simulink model "Mode_AAI"  (R2022b)
settings: Solver=FixedStepAuto  StartTime=0.0  StopTime=10.0  FixedStep=1e-3  RelTol=1e-3  EnableMultiTasking=on
undefined symbols (not defined in the file): D0, D10, D11, D12, D13, D2, D4, D5, D6, D7, D8, D9, PTA0, PTA2, PTB23, PTB9, PTC16, PTC2, PTC3, PTC4, PTD0, PTD1, PTD2, PTD3
libraries: frdmk64flib x14
settings Model: ExtModeTrigDuration=5  Creator=sarahalabdulrazzak  LastModifiedBy=kavem
settings SolverCC: AlgebraicLoopSolver=TrustRegion
settings OptimizationCC: EnhancedBackFolding=on  PassReuseOutputArgsAs=Individual arguments  ZeroExternalMemoryAtStartup=off  ZeroInternalMemoryAtStartup=off  MaxStackSize=64  OptimizeBlockOrder=speed  DifferentSizesBufferReuse=on  OptimizationCustomize=off  EfficientTunableParamExpr=on
settings DebuggingCC: ParameterTunabilityLossMsg=error  UnconnectedInputMsg=warning  UnconnectedOutputMsg=warning  UnconnectedLineMsg=warning  SFMachineParentedDataDiag=warning
settings HardwareCC: ProdBitPerPointer=32  ProdBitPerSizeT=32  ProdBitPerPtrDiffT=32  ProdLargestAtomicInteger=Long  ProdLargestAtomicFloat=Double  ProdWordSize=32  ProdHWDeviceType=ARM Compatible->ARM Cortex
settings ModelReferenceCC: EnableRefExpFcnMdlSchedulingChecks=on
settings SFSimCC: MATLABDynamicMemAlloc=off
settings RTWCC: Description=Embedded Coder  SystemTargetFile=ert.tlc  HardwareBoard=NXP FRDM-K64F  TLCOptions="-aInlineSetEventsForThisBaseRateFcn=TLC_FALSE -aSuppressMultiTaskScheduler=TLC_FALSE  -aRateBasedStepFcn=0"  TemplateMakefile=ert_default_tmf  Toolchain=GNU Tools for ARM Embedded Processors
settings CodeAppCC: ForceParamTrailComments=on  IgnoreCustomStorageClasses=off  OperatorAnnotations=on  SimulinkDataObjDesc=on  SFDataObjDesc=on  InsertBlockDesc=on

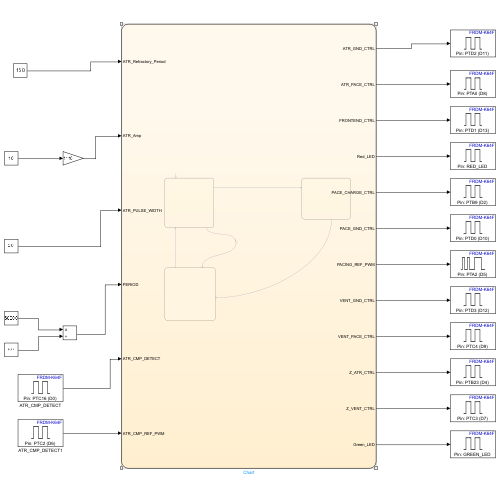
[thumbnail: Simulink's stored preview of the top-level diagram]
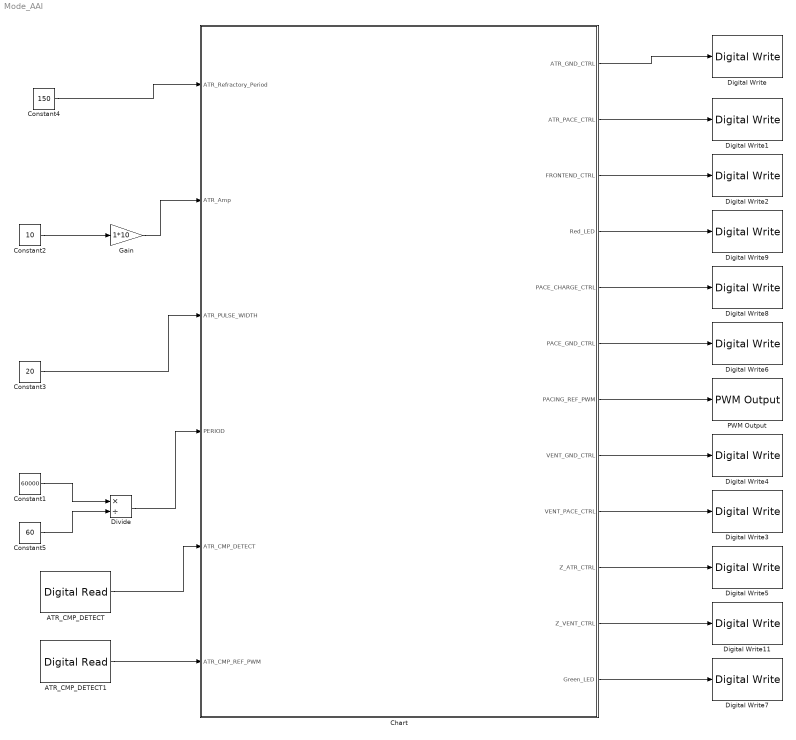
== system Mode_AAI ==
  ATR_CMP_DETECT : frdmk64flib/Digital Read  Whichpin=PTC16 (D0)  SampleTime=-1
  ATR_CMP_DETECT1 : frdmk64flib/Digital Read  Whichpin=PTC2 (D6)  SampleTime=-1
  Chart : Stateflow chart  TreatAsAtomicUnit=on
  Constant1 : Constant  Value=60000
  Constant2 : Constant  Value=10
  Constant3 : Constant  Value=20
  Constant4 : Constant  Value=150
  Constant5 : Constant  Value=60
  Digital Write : frdmk64flib/Digital Write  Whichpin=PTD2 (D11)
  Digital Write1 : frdmk64flib/Digital Write  Whichpin=PTA0 (D8)
  Digital Write11 : frdmk64flib/Digital Write  Whichpin=PTC3 (D7)
  Digital Write2 : frdmk64flib/Digital Write  Whichpin=PTD1 (D13)
  Digital Write3 : frdmk64flib/Digital Write  Whichpin=PTC4 (D9)
  Digital Write4 : frdmk64flib/Digital Write  Whichpin=PTD3 (D12)
  Digital Write5 : frdmk64flib/Digital Write  Whichpin=PTB23 (D4)
  Digital Write6 : frdmk64flib/Digital Write  Whichpin=PTD0 (D10)
  Digital Write7 : frdmk64flib/Digital Write  Whichpin=GREEN_LED
  Digital Write8 : frdmk64flib/Digital Write  Whichpin=PTB9 (D2)
  Digital Write9 : frdmk64flib/Digital Write  Whichpin=RED_LED
  Divide : Product  Inputs=*/
  Gain : Gain  Gain=1*10
  PWM Output : frdmk64flib/PWM Output  Whichpin=PTA2 (D5)  InitialFrequency=2000  InitialDutyCycle=0
  wires:
  Constant3/1 -> Chart/3(ATR_PULSE_WIDTH)
  Constant4/1 -> Chart/1(ATR_Refractory_Period)
  Chart/1(ATR_GND_CTRL) -> Digital Write/1
  Chart/2(ATR_PACE_CTRL) -> Digital Write1/1
  Chart/3(FRONTEND_CTRL) -> Digital Write2/1
  Chart/4(Red_LED) -> Digital Write9/1
  Chart/5(PACE_CHARGE_CTRL) -> Digital Write8/1
  Chart/6(PACE_GND_CTRL) -> Digital Write6/1
  Chart/7(PACING_REF_PWM) -> PWM Output/1
  Chart/8(VENT_GND_CTRL) -> Digital Write4/1
  Chart/9(VENT_PACE_CTRL) -> Digital Write3/1
  Chart/10(Z_ATR_CTRL) -> Digital Write5/1
  Chart/11(Z_VENT_CTRL) -> Digital Write11/1
  Constant5/1 -> Divide/2
  Constant1/1 -> Divide/1
  Divide/1 -> Chart/4(PERIOD)
  Constant2/1 -> Gain/1
  Gain/1 -> Chart/2(ATR_Amp)
  ATR_CMP_DETECT/1 -> Chart/5(ATR_CMP_DETECT)
  Chart/12(Green_LED) -> Digital Write7/1
  ATR_CMP_DETECT1/1 -> Chart/6(ATR_CMP_REF_PWM)

== stateflow chart Mode_AAI/Chart ==
  state CHARGING
    entry:
    %sensing ON
    FRONTEND_CTRL = HIGH
    %Charge primary capcitor C22
    ATR_PACE_CTRL=LOW
    VENT_PACE_CTRL=LOW
    PACING_REF_PWM = ATR_Amp
    PACE_CHARGE_CTRL = HIGH
    %Discharge block capacitor C21
    PACE_GND_CTRL = HIGH
    VENT_PACE_CTRL = LOW
    Z_ATR_CTRL = LOW
    Z_VENT_CTRL = LOW
    ATR_GND_CTRL = HIGH
    VENT_GND_CTRL = LOW
    %use LED  to verify state
    Red_LED=false
    Green_LED=true
  state DISCHARGING
    %sensing OFF
    FRONTEND_CTRL = LOW
    %Discharge C22 primary capacitor
    %Charge C21 block capacitor
    PACE_CHARGE_CTRL = LOW
    PACE_GND_CTRL = HIGH
    ATR_PACE_CTRL = HIGH
    ATR_GND_CTRL = LOW
    Z_ATR_CTRL = LOW
    Z_VENT_CTRL = LOW
    VENT_GND_CTRL = LOW
    VENT_PACE_CTRL  = LOW
    PACING_REF_PWM = ATR_Amp
    %use LED  to verify state
    Red_LED=true
  state STATE
    entry:
    %sensing ON
    FRONTEND_CTRL = LOW
    %Charge primary capcitor C22
    ATR_PACE_CTRL=LOW
    VENT_PACE_CTRL=LOW
    PACING_REF_PWM = ATR_Amp
    PACE_CHARGE_CTRL = HIGH
    %Discharge block capacitor C21
    PACE_GND_CTRL = HIGH
    VENT_PACE_CTRL = LOW
    Z_ATR_CTRL = LOW
    Z_VENT_CTRL = LOW
    ATR_GND_CTRL = HIGH
    VENT_GND_CTRL = LOW
    %use LED  to verify state
    Red_LED=false
    Green_LED=false
  (default) -> CHARGING
  CHARGING -> DISCHARGING [order 1] : after(PERIOD - ATR_PULSE_WIDTH,msec)
  DISCHARGING -> STATE : after(ATR_PULSE_WIDTH, msec)
  STATE -> CHARGING : after(ATR_Refractory_Period,msec)
  CHARGING -> (junction 67) [order 2] : [ATR_CMP_DETECT==true]
  (junction 67) -> STATE : after(ATR_PULSE_WIDTH,msec)
  data: ATR_Refractory_Period input; ATR_Amp input; ATR_GND_CTRL output; ATR_PACE_CTRL output; FRONTEND_CTRL output; Red_LED output; PACE_CHARGE_CTRL output; PACE_GND_CTRL output; PACING_REF_PWM output; VENT_GND_CTRL output; VENT_PACE_CTRL output; Z_ATR_CTRL output; Z_VENT_CTRL output; ATR_PULSE_WIDTH input; HIGH local =true; LOW local =false; PERIOD input; ATR_CMP_DETECT input; Green_LED output; ATR_CMP_REF_PWM input
